simulink model "RollControlSimulation"  (R2021a)
settings: Solver=VariableStepAuto  StartTime=0.0  StopTime=200  RelTol=1e-3
values from neighbouring files (symbols this model uses):
  Ar = pi*radius^2    (= 0.00879146429773)    [RollControlParameters.m]
  C = derivada_coef_D_aletas + derivada_coef_D_canards    (= 37.955768493)    [RollControlParameters.m]
  derivada_coef_f_aletas = 10.88468582071296    (= 10.8846858207)    [RollControlParameters.m]
  derivada_coef_f_canards = 1.6496306282951438    (= 1.6496306283)    [RollControlParameters.m]
  DynamicPressure = (speed^2)*rho/2    (= 9976.6352)    [RollControlParameters.m]
  J = 0.030    (= 0.03)    [RollControlParameters.m]
  Lr = 2*radius    (= 0.1058)    [RollControlParameters.m]
  P = DynamicPressure * Ar * Lr * Lr / 2 / speed    (= 0.00357793574932)    [RollControlParameters.m]
  tau_s = 0.07/(pi/3)    (= 0.0668450760986)    [RollControlParameters.m]
libraries: dspsrcs4 x1, slpidlib x1, simulink x1
settings Model: Creator=wujia  LastModifiedBy=wujia
settings OptimizationCC: ZeroExternalMemoryAtStartup=off  ZeroInternalMemoryAtStartup=off
settings RTWCC: TargetLang=C++
settings GRTTargetCC: TargetLangStandard=C++03 (ISO)  CodeInterfacePackaging=C++ class

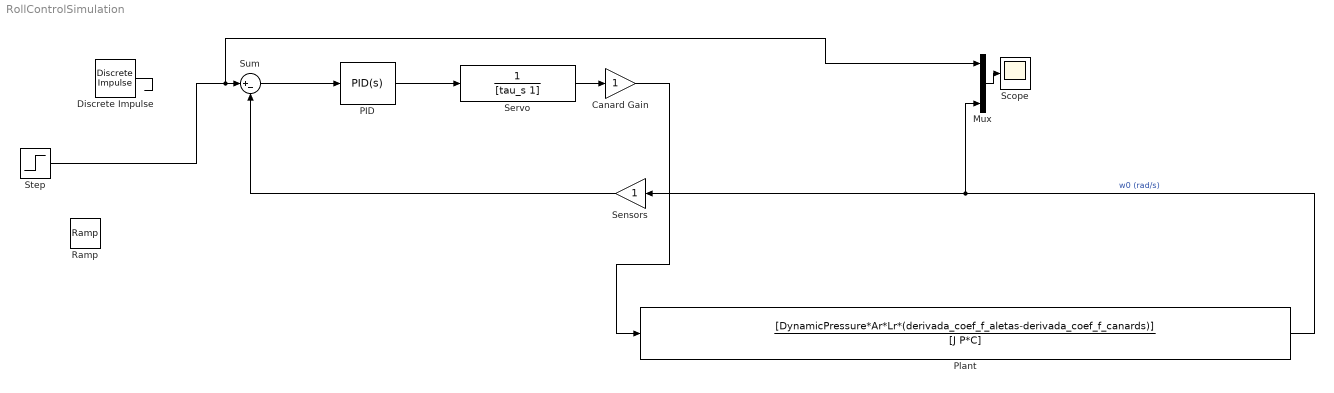
== system RollControlSimulation ==
  Canard Gain : Gain
  Discrete Impulse : dspsrcs4/Discrete  Impulse  Delay=0  SampleTime=1  FrameSample=1  OutputFrames=off  dataType=double  isSigned=on  wordLen=16  udDataType=sfix(16)  fracBitsMode=Best precision  numFracBits=15  OutDataTypeStr=double  LastOutDataTypeStr=double
  Mux : Mux  Inputs=3
  PID : slpidlib/PID Controller  Controller=PID  Form=Ideal  TimeDomain=Continuous-time  UseExternalTs=off  SampleTime=-1  IntegratorMethod=Forward Euler  FilterMethod=Forward Euler  ControllerParametersSource=internal  P=0.00415792267673615  I=10.82837532756  D=0.00111895618386219  UseFilter=on  N=14.0446272815803  TunerSelectOption=Transfer Function Based (PID Tuner App)  InitialConditionSource=internal  InitialConditionForIntegrator=0  InitialConditionForFilter=0  DifferentiatorICPrevScaledInput=0  ExternalReset=none  TrackingMode=off  Kt=1  LimitOutput=on  SatLimitsSource=internal  UpperSaturationLimit=8  LowerSaturationLimit=-8  LinearizeAsGain=on  AntiWindupMode=clamping  Kb=1  POutMin=[]  POutMax=[]  IOutMin=[]  IOutMax=[]  DOutMin=[]  DOutMax=[]  NOutMin=[]  NOutMax=[]  SumOutMin=[]  SumOutMax=[]  SaturationOutMin=[]  SaturationOutMax=[]  PParamMin=[]  PParamMax=[]  IParamMin=[]  IParamMax=[]  DParamMin=[]  DParamMax=[]  NParamMin=[]  NParamMax=[]  KbParamMin=[]  KbParamMax=[]  KtParamMin=[]  KtParamMax=[]  KbOutMin=[]  KbOutMax=[]  KtOutMin=[]  KtOutMax=[]  IntegratorOutMin=[]  IntegratorOutMax=[]  FilterOutMin=[]  FilterOutMax=[]  SumI1OutMin=[]  SumI1OutMax=[]  SumI2OutMin=[]  SumI2OutMax=[]  SumI3OutMin=[]  SumI3OutMax=[]  SumI4OutMin=[]  SumI4OutMax=[]  SumDOutMin=[]  SumDOutMax=[]  DifferentiatorOutMin=[]  DifferentiatorOutMax=[]  FilterDiffOutCoefMin=[]  FilterDiffOutCoefMax=[]  ReciprocalOutMin=[]  ReciprocalOutMax=[]  SumDenOutMin=[]  SumDenOutMax=[]  SumNumOutMin=[]  SumNumOutMax=[]  DivideOutMin=[]  DivideOutMax=[]  UdiffTsProdOutMin=[]  UdiffTsProdOutMax=[]  NTsProdOutMin=[]  NTsProdOutMax=[]  UintegralTsProdOutMin=[]  UintegralTsProdOutMax=[]  UngainTsProdOutMin=[]  UngainTsProdOutMax=[]  IntegratorContinuousStateAttributes=''  IntegratorStateMustResolveToSignalObject=off  IntegratorRTWStateStorageClass=Auto  FilterContinuousStateAttributes=''  FilterStateMustResolveToSignalObject=off  FilterRTWStateStorageClass=Auto  ParallelPVariant=Passthrough  IdealPVariant=InternalParameters  IVariant=InternalParameters  DVariant=InternalParameters  IntegratorVariant=Continuous  SatVariant=Enabled  AWVariant=ContClampingIdeal  PCopyVariant=InternalParamsIdeal  TRVariant=Disabled  FdbkBlocksVariant=Forward  IdealPFdbkVariant=Disabled  SatFdbkVariant=Disabled  DerivativeFilterVariant=ContFilter  NVariant=InternalParameters  NCopyVariant=Disabled  FilterICVariant=InternalICsFilter  IntegratorICVariant=InternalICs  ExternalResetVariant=Disabled  TRSumVariant=Passthrough  SumFdbkVariant=Disabled  SumVariant=Sum_PID  TsampFilterVariant=InternalTs  TsampNgainVariant=Passthrough  TsampIntegralVariant=Passthrough  ExternalSaturationOutDataTypeStr=Inherit: Same as second input
  Plant : TransferFcn  Numerator=[DynamicPressure*Ar*Lr*(derivada_coef_f_aletas-derivada_coef_f_canards)]  Denominator=[J P*C]
  Ramp : simulink/Sources/Ramp  slope=0.2  start=0  InitialOutput=0
  Scope : Scope
  Sensors : Gain
  Servo : TransferFcn  Denominator=[tau_s 1]
  Step : Step  Time=100  Before=10  After=0  SampleTime=0
  Sum : Sum  Inputs=|+-
  wires:
  Sensors/1 -> Sum/2
  Canard Gain/1 -> Plant/1
  Mux/1 -> Scope/1
  Sum/1 -> PID/1
  PID/1 -> Servo/1
  Plant/1 -> Mux/3, Sensors/1  "w0 (rad/s)"
  Servo/1 -> Canard Gain/1
  Discrete Impulse/1 -> ?
  Step/1 -> Mux/1, Sum/1
